simulink model "TPTC_Vehicle_dynamics_pedal2torque_NeglectSOC"  (R2026a)
settings: Solver=ode23tb  StopTime=40
model workspace (MAT data in the model file):
  BattChrgMax = -500000
  BattDischrgMax = 500000
  ChrgLmt_bpt = [1 1 1 1 1 1 1 1 0.7 0.35 0]
  DischrgLmt_bpt = [0 0.35 0.7 1 1 1 1 1 1 1 1]
  SOC_bpt = [0 10 20 30 40 50 60 70 80 90 100]
  motorMaxTorqueNm = [500 500 500 500 500 500 416.666666667 357.142857143 312.5 277.777777778 250 227.272727273 ... (16 elements, 1x16)]
  motorSpeedRadPs = [0 40 80 120 160 200 240 280 320 360 400 440 ... (16 elements, 1x16)]
values from neighbouring files (symbols this model uses):
  alpha_thr = Simulink.Parameter(300)    [init_MCU_ASR_params_only.m]
  eta_drv = Simulink.Parameter(0.95)    [init_MCU_ASR_params_only.m]
  gear_ratio_F = Simulink.Parameter(10.91)    [init_MCU_ASR_params_only.m]
  gear_ratio_R = Simulink.Parameter(11.62)    [init_MCU_ASR_params_only.m]
  J_axle = Simulink.Parameter(2*I_tire)    [init_MCU_ASR_params_only.m]
  Kd_damp = Simulink.Parameter(0.025)    [init_MCU_ASR_params_only.m]
  R_tire = Simulink.Parameter(r)    [init_MCU_ASR_params_only.m]
  T_active = Simulink.Parameter(15)    [init_MCU_ASR_params_only.m]
  T_damp_lim = Simulink.Parameter(18)    [init_MCU_ASR_params_only.m]
  tau_lpf_damp = Simulink.Parameter(0.060)    [init_MCU_ASR_params_only.m]
  Tlim_down_rate = Simulink.Parameter(2000)    [init_MCU_ASR_params_only.m]
  Tlim_up_rate = Simulink.Parameter(120)    [init_MCU_ASR_params_only.m]
  Tlim_warn_rate = Simulink.Parameter(600)    [init_MCU_ASR_params_only.m]
  Tmax_mot = Simulink.Parameter(Tn_motor)    [init_MCU_ASR_params_only.m]
  Ts_asr = Simulink.Parameter(0.001)    [init_MCU_ASR_params_only.m]
undefined symbols (not defined in the file or in its folder): dspblkCoreblockFVToolHelper, gcbh, gear_ratio
libraries: autolibsharedcoupling x8, simulink x3, autolibshareddiff x2, autolibmappedmotor x2, slpidlib x1, autolibdatasheetbattery x1, sim3dlib x1, sim3dautolib x1, vehdynlibsteering x1
(part 4 of 4)

== matlab function TPTC_Vehicle_dynamics_pedal2torque_NeglectSOC/Powertrain/03_MCU_TPTC_Controller/Slip_Detector_Front/MATLAB Function ==
  data: Te input; risk output; warn output; alpha input; Tload input; omega input; Te_opp input; alpha_opp input; Tload_opp input; omega_opp input; T_active input; alpha_thr input; state output; Ts input; Treq input; load_ratio output; follow_bad output; axis_diverge output; startup_guard output; limit_ratio output
function [risk,warn,state,load_ratio,follow_bad,...
    axis_diverge,startup_guard,limit_ratio] = f( ...
    Te,alpha,Tload,omega, ...
    Te_opp,alpha_opp,Tload_opp,omega_opp, ...
    T_active,alpha_thr,Ts,Treq)
%#codegen

% ============================================================
% MCU级 TPTC/ASR 滑移风险检测状态机
%
% 不使用滑移率，不使用车辆纵向速度。
%
% 输入：
%   Te          本轴实际/估算电机扭矩，N*m
%   alpha       本轴电机机械角加速度，rad/s^2
%   Tload       本轴电机侧负载转矩观测值，N*m
%   omega       本轴电机机械角速度，rad/s
%
%   Te_opp      对轴电机扭矩，N*m
%   alpha_opp   对轴电机角加速度，rad/s^2
%   Tload_opp   对轴负载转矩观测值，N*m
%   omega_opp   对轴电机机械角速度，rad/s
%
%   T_active    有效驱动请求阈值，N*m
%   alpha_thr   基础角加速度阈值，rad/s^2
%   Ts          控制周期，s
%   Treq        限扭前VCU目标扭矩，N*m
%
% 输出：
%   risk           Risk标志
%   warn           Warning标志
%   state          0 Normal / 1 Warning / 2 Risk
%   load_ratio     当前负载支持能力，正常约为1
%   follow_bad     负载传递异常
%   axis_diverge   前后轴动态分化诊断
%   startup_guard  起步保护标志
%   limit_ratio    目标限扭比例
%
% 状态控制：
%   Normal  ：limit_ratio = 1.00
%   Warning ：limit_ratio = 0.82
%   Risk    ：limit_ratio = 0.50~0.70，自适应
%
% 关键修改：
%   1. 持续严重负载缺失可以直接进入Risk；
%   2. 不再强制要求Risk必须伴随明显alpha异常；
%   3. Warning状态真正执行82%轻度限扭；
%   4. Warning期间负载能力仍严重不足时升级Risk；
%   5. Risk/Warning期间冻结正常负载基线；
%   6. 进入和退出均设置计数确认，避免抖振。
% ============================================================


%% ============================================================
% 1. 持久变量
% =============================================================

persistent initialized
persistent state_z

persistent active_cnt
persistent baseline_cnt
persistent baseline_valid
persistent cooldown_cnt

persistent q_fast_z
persistent q_ref_z
persistent q_rate_z

persistent omega_z
persistent omega_opp_z

persistent risk_enter_cnt
persistent warn_enter_cnt
persistent risk_reenter_cnt
persistent severe_load_cnt

persistent state_hold_cnt
persistent stable_cnt

persistent risk_ratio_z


%% ============================================================
% 2. 初始化
% =============================================================

if isempty(initialized)

    state_z = 0.0;

    active_cnt = 0.0;
    baseline_cnt = 0.0;
    baseline_valid = false;
    cooldown_cnt = 0.0;

    q_fast_z = 0.0;
    q_ref_z = 0.0;
    q_rate_z = 0.0;

    omega_z = 0.0;
    omega_opp_z = 0.0;

    risk_enter_cnt = 0.0;
    warn_enter_cnt = 0.0;
    risk_reenter_cnt = 0.0;
    severe_load_cnt = 0.0;

    state_hold_cnt = 0.0;
    stable_cnt = 0.0;

    risk_ratio_z = 0.60;

    initialized = true;
end


%% ============================================================
% 3. 采样周期和输入保护
% =============================================================

if Ts > 0.0
    Ts_eff = Ts;
else
    Ts_eff = 1.0e-3;
end

T_active_eff = max(abs(T_active),1.0);
alpha_thr_eff = max(abs(alpha_thr),1.0);

Treq_abs = abs(Treq);
Te_abs = abs(Te);
Tload_abs = abs(Tload);


%% ============================================================
% 4. 统一角加速度方向
%
% alpha_drv > 0表示电机转速幅值增加。
% =============================================================

drive_dir = 1.0;

if abs(omega) > 1.0

    if omega < 0.0
        drive_dir = -1.0;
    end

elseif Te_abs > 1.0

    if Te < 0.0
        drive_dir = -1.0;
    end
end

alpha_drv = drive_dir*alpha;


drive_dir_opp = 1.0;

if abs(omega_opp) > 1.0

    if omega_opp < 0.0
        drive_dir_opp = -1.0;
    end

elseif abs(Te_opp) > 1.0

    if Te_opp < 0.0
        drive_dir_opp = -1.0;
    end
end

alpha_opp_drv = drive_dir_opp*alpha_opp;


%% ============================================================
% 5. 标定参数
% =============================================================

% 起步保护
startup_guard_time = 0.050;
initial_blank_time = 0.050;

startup_guard_steps = ...
    max(1.0,ceil(startup_guard_time/Ts_eff));

initial_blank_steps = ...
    max(1.0,ceil(initial_blank_time/Ts_eff));


% 正常负载基线学习时间
baseline_learn_time = 0.400;

baseline_learn_steps = ...
    max(1.0,ceil(baseline_learn_time/Ts_eff));


% 回到Normal后的检测冷却时间
cooldown_time = 0.300;

cooldown_steps = ...
    max(1.0,ceil(cooldown_time/Ts_eff));


% Normal状态进入确认
risk_enter_time = 0.008;
warn_enter_time = 0.020;

risk_enter_steps = ...
    max(1.0,ceil(risk_enter_time/Ts_eff));

warn_enter_steps = ...
    max(1.0,ceil(warn_enter_time/Ts_eff));


% Warning重新升级Risk确认
risk_reenter_time = 0.020;

risk_reenter_steps = ...
    max(1.0,ceil(risk_reenter_time/Ts_eff));


% 持续严重负载不足确认
severe_load_time = 0.030;

severe_load_steps = ...
    max(1.0,ceil(severe_load_time/Ts_eff));


% Risk保持和退出确认
risk_hold_time = 0.250;
risk_stable_time = 0.200;

risk_hold_steps = ...
    max(1.0,ceil(risk_hold_time/Ts_eff));

risk_stable_steps = ...
    max(1.0,ceil(risk_stable_time/Ts_eff));


% Warning保持和退出确认
warn_hold_time = 0.300;
warn_stable_time = 0.300;

warn_hold_steps = ...
    max(1.0,ceil(warn_hold_time/Ts_eff));

warn_stable_steps = ...
    max(1.0,ceil(warn_stable_time/Ts_eff));


% 负载指标滤波
tau_q_fast = 0.030;
tau_q_ref = 1.500;
tau_q_rate = 0.030;

a_q_fast = ...
    Ts_eff/(tau_q_fast + Ts_eff);

a_q_ref = ...
    Ts_eff/(tau_q_ref + Ts_eff);

a_q_rate = ...
    Ts_eff/(tau_q_rate + Ts_eff);


% Normal状态负载阈值
q_warn_thr = 0.85;
q_risk_thr = 0.68;
q_dynamic_thr = 0.78;

% 严重负载支持能力阈值
severe_load_thr = 0.72;

% 相对负载下降速率阈值，单位1/s
q_rate_warn_thr = -0.30;
q_rate_risk_thr = -0.70;


% Risk恢复到Warning
support_risk_recover_thr = 0.80;

% Warning恢复期间重新恶化
support_reenter_thr = 0.72;

% Warning退出到Normal
support_normal_thr = 0.88;


% 角加速度阈值
alpha_warn_thr = 0.55*alpha_thr_eff;
alpha_risk_thr = 0.85*alpha_thr_eff;
alpha_strong_thr = 1.25*alpha_thr_eff;


% 限扭比例
warning_limit_ratio = 0.82;

risk_ratio_min = 0.50;
risk_ratio_max = 0.70;
risk_ratio_margin = 0.10;


% 前后轴分化阈值，仅作诊断
alpha_diff_thr = 0.60*alpha_thr_eff;
omega_diff_thr = 10.0;
omega_diff_rate_thr = 80.0;


%% ============================================================
% 6. 有效驱动请求判断
%
% 必须使用限扭前Treq。
% =============================================================

active = (Treq_abs > T_active_eff);

if active

    active_cnt = active_cnt + 1.0;

else

    active_cnt = 0.0;

    state_z = 0.0;

    baseline_cnt = 0.0;
    baseline_valid = false;
    cooldown_cnt = 0.0;

    risk_enter_cnt = 0.0;
    warn_enter_cnt = 0.0;
    risk_reenter_cnt = 0.0;
    severe_load_cnt = 0.0;

    state_hold_cnt = 0.0;
    stable_cnt = 0.0;

    risk_ratio_z = 0.60;
end

startup_guard = ...
    active && (active_cnt <= startup_guard_steps);

initial_blank = ...
    active && (active_cnt <= initial_blank_steps);


%% ============================================================
% 7. 实际扭矩执行比例
% =============================================================

if Treq_abs > 1.0

    torque_ratio_applied = ...
        Te_abs/Treq_abs;

else

    torque_ratio_applied = 0.0;
end

if torque_ratio_applied < 0.0

    torque_ratio_applied = 0.0;

elseif torque_ratio_applied > 1.20

    torque_ratio_applied = 1.20;
end


%% ============================================================
% 8. 负载观测有效性
% =============================================================

observer_valid = ...
    active && ...
    (Te_abs > max(0.20*Treq_abs,...
                  0.50*T_active_eff));


%% ============================================================
% 9. 负载指标
%
% q = |Tload_hat|/|Treq|
%
% 使用限扭前请求作分母，避免限扭动作直接改变分母。
% =============================================================

q_raw = ...
    Tload_abs/max(Treq_abs,1.0);

if q_raw < 0.0

    q_raw = 0.0;

elseif q_raw > 2.50

    q_raw = 2.50;
end


%% ============================================================
% 10. 当前负载快速滤波及变化率
% =============================================================

if ~active

    q_fast_z = q_raw;
    q_ref_z = q_raw;
    q_rate_z = 0.0;

elseif observer_valid

    if active_cnt <= 1.0

        q_fast_z = q_raw;
        q_ref_z = q_raw;
        q_rate_z = 0.0;

    else

        q_fast_old = q_fast_z;

        q_fast_z = ...
            q_fast_z + ...
            a_q_fast*(q_raw-q_fast_z);

        q_rate_raw = ...
            (q_fast_z-q_fast_old)/Ts_eff;

        q_rate_z = ...
            q_rate_z + ...
            a_q_rate*(q_rate_raw-q_rate_z);
    end

else

    % 观测无效时，变化率缓慢回零
    q_rate_z = ...
        q_rate_z + ...
        a_q_rate*(0.0-q_rate_z);
end


%% ============================================================
% 11. 冷却计数
% =============================================================

if cooldown_cnt > 0.0
    cooldown_cnt = cooldown_cnt-1.0;
end


%% ============================================================
% 12. 正常负载基线学习
%
% 只允许在：
%   Normal、基本全扭矩、动态稳定时更新。
% Warning/Risk期间冻结。
% =============================================================

normal_baseline_condition = ...
    active && ...
    observer_valid && ...
    (state_z == 0.0) && ...
    (torque_ratio_applied > 0.92) && ...
    (abs(alpha_drv) < 0.35*alpha_thr_eff);


if normal_baseline_condition

    if ~baseline_valid

        baseline_cnt = baseline_cnt + 1.0;

        if baseline_cnt <= 1.0

            q_ref_z = q_fast_z;

        else

            q_ref_z = ...
                q_ref_z + ...
                a_q_ref*(q_fast_z-q_ref_z);
        end

        if baseline_cnt >= baseline_learn_steps
            baseline_valid = true;
        end

    else

        q_ref_pre = max(q_ref_z,0.02);

        q_full_pre = ...
            q_fast_z/q_ref_pre;

        q_rate_pre = ...
            q_rate_z/q_ref_pre;

        normal_for_update = ...
            (q_full_pre > 0.90) && ...
            (q_full_pre < 1.12) && ...
            (abs(q_rate_pre) < 0.12);

        if normal_for_update

            q_ref_z = ...
                q_ref_z + ...
                a_q_ref*(q_fast_z-q_ref_z);
        end
    end
end


%% ============================================================
% 13. 负载能力指标
%
% q_full：
%   当前负载相对全扭矩正常基线的比例。
%
% q_support：
%   对当前限扭比例补偿后的负载支持能力。
% =============================================================

if baseline_valid

    q_ref_den = max(q_ref_z,0.02);

    q_full = ...
        q_fast_z/q_ref_den;

    q_rate_rel = ...
        q_rate_z/q_ref_den;

    applied_ratio_den = ...
        max(torque_ratio_applied,0.20);

    q_support = ...
        q_fast_z/...
        (q_ref_den*applied_ratio_den);

else

    q_full = 1.0;
    q_rate_rel = 0.0;
    q_support = 1.0;
end


if q_full < 0.0

    q_full = 0.0;

elseif q_full > 3.0

    q_full = 3.0;
end


if q_support < 0.0

    q_support = 0.0;

elseif q_support > 3.0

    q_support = 3.0;
end


% 对外输出当前扭矩水平下的负载支持能力
load_ratio = q_support;


%% ============================================================
% 14. Normal状态检测器使能
% =============================================================

detector_armed = ...
    baseline_valid && ...
    active && ...
    (state_z == 0.0) && ...
    (cooldown_cnt <= 0.0) && ...
    (torque_ratio_applied > 0.90);


%% ============================================================
% 15. 一般负载异常判据
% =============================================================

load_low_warn = ...
    detector_armed && ...
    (q_full < q_warn_thr);

load_low_risk = ...
    detector_armed && ...
    (q_full < q_risk_thr);

load_drop_warn = ...
    detector_armed && ...
    (q_rate_rel < q_rate_warn_thr);

load_drop_risk = ...
    detector_armed && ...
    (q_rate_rel < q_rate_risk_thr);


%% ============================================================
% 16. 持续严重负载能力不足
%
% Normal使用q_full。
% Warning使用补偿限扭影响后的q_support。
%
% 该路径不强制要求alpha异常，用于解决：
% 开式差速器单轮空转被电机平均转速掩盖的问题。
% =============================================================

if state_z == 0.0

    severe_load_metric = q_full;

    severe_load_enable = ...
        detector_armed && ...
        (torque_ratio_applied > 0.90);

elseif state_z == 1.0

    severe_load_metric = q_support;

    severe_load_enable = ...
        active && ...
        observer_valid && ...
        (torque_ratio_applied > 0.50);

else

    severe_load_metric = q_support;
    severe_load_enable = false;
end


severe_load_raw = ...
    severe_load_enable && ...
    (severe_load_metric < severe_load_thr);


if severe_load_raw

    severe_load_cnt = severe_load_cnt + 1.0;

    if severe_load_cnt > severe_load_steps
        severe_load_cnt = severe_load_steps;
    end

else

    severe_load_cnt = 0.0;
end


severe_load_confirmed = ...
    (severe_load_cnt >= severe_load_steps);


follow_bad = ...
    load_low_warn || ...
    load_drop_warn || ...
    severe_load_confirmed || ...
    ( ...
      (state_z ~= 0.0) && ...
      (q_support < support_risk_recover_thr) ...
    );


%% ============================================================
% 17. 电机角加速度条件
% =============================================================

alpha_warn = ...
    (alpha_drv > alpha_warn_thr);

alpha_risk = ...
    (alpha_drv > alpha_risk_thr);

alpha_strong = ...
    (alpha_drv > alpha_strong_thr);


%% ============================================================
% 18. 前后轴动态分化诊断
%
% 当前仅输出诊断，不直接决定状态。
% =============================================================

omega_diff = ...
    abs(omega)-abs(omega_opp);

omega_diff_old = ...
    abs(omega_z)-abs(omega_opp_z);

d_omega_diff = ...
    (omega_diff-omega_diff_old)/Ts_eff;


alpha_diverge = ...
    (~startup_guard) && ...
    alpha_warn && ...
    (alpha_drv > ...
     alpha_opp_drv+alpha_diff_thr);


omega_diverge = ...
    (~startup_guard) && ...
    (omega_diff > omega_diff_thr) && ...
    (d_omega_diff > omega_diff_rate_thr);


axis_diverge = ...
    alpha_diverge || omega_diverge;


%% ============================================================
% 19. Normal状态进入条件
% =============================================================

risk_enter_raw = false;
warn_enter_raw = false;

if state_z == 0.0 && ...
        active && ...
        (~initial_blank)

    % 路径1：负载严重降低并伴随动态异常
    risk_path_main = ...
        load_low_risk && ...
        (alpha_risk || load_drop_risk);

    % 路径2：负载中度降低且快速恶化
    risk_path_dynamic = ...
        detector_armed && ...
        (q_full < q_dynamic_thr) && ...
        load_drop_risk && ...
        alpha_warn;

    % 路径3：极强角加速度且负载已经下降
    risk_path_strong = ...
        detector_armed && ...
        alpha_strong && ...
        (q_full < 0.90);

    % 路径4：持续严重负载不足
    % 不要求alpha必须明显异常
    risk_path_sustained_load = ...
        severe_load_confirmed;

    risk_enter_raw = ...
        risk_path_main || ...
        risk_path_dynamic || ...
        risk_path_strong || ...
        risk_path_sustained_load;


    % Warning：中度负载异常
    warn_path_main = ...
        load_low_warn && ...
        (alpha_warn || load_drop_warn);

    warn_enter_raw = ...
        warn_path_main;
end


% Risk优先
if risk_enter_raw
    warn_enter_raw = false;
end


%% ============================================================
% 20. Normal状态进入确认计数
% =============================================================

if risk_enter_raw

    risk_enter_cnt = risk_enter_cnt + 1.0;

    if risk_enter_cnt > risk_enter_steps
        risk_enter_cnt = risk_enter_steps;
    end

else

    risk_enter_cnt = 0.0;
end


if warn_enter_raw

    warn_enter_cnt = warn_enter_cnt + 1.0;

    if warn_enter_cnt > warn_enter_steps
        warn_enter_cnt = warn_enter_steps;
    end

else

    warn_enter_cnt = 0.0;
end


risk_enter = ...
    (risk_enter_cnt >= risk_enter_steps);

warn_enter = ...
    (warn_enter_cnt >= warn_enter_steps);


%% ============================================================
% 21. Warning重新升级Risk
%
% 满足任一条件：
%   1. 极强角加速度；
%   2. 持续严重负载能力不足；
%   3. 负载支持能力低且角加速度异常。
% =============================================================

risk_reenter_raw = ...
    (state_z == 1.0) && ...
    active && ...
    ( ...
      alpha_strong || ...
      severe_load_confirmed || ...
      ( ...
        (q_support < support_reenter_thr) && ...
        alpha_warn ...
      ) ...
    );


if risk_reenter_raw

    risk_reenter_cnt = risk_reenter_cnt + 1.0;

    if risk_reenter_cnt > risk_reenter_steps
        risk_reenter_cnt = risk_reenter_steps;
    end

else

    risk_reenter_cnt = 0.0;
end


risk_reenter = ...
    (risk_reenter_cnt >= risk_reenter_steps);


%% ============================================================
% 22. 三状态状态机
% =============================================================

if ~active

    % --------------------------------------------------------
    % 无驱动请求
    % --------------------------------------------------------

    state_z = 0.0;

    state_hold_cnt = 0.0;
    stable_cnt = 0.0;


elseif state_z == 0.0

    % --------------------------------------------------------
    % Normal
    % --------------------------------------------------------

    state_hold_cnt = 0.0;
    stable_cnt = 0.0;

    if risk_enter

        % 根据检测时负载能力确定Risk限扭比例
        ratio_candidate = ...
            q_full+risk_ratio_margin;

        if ratio_candidate < risk_ratio_min

            risk_ratio_z = risk_ratio_min;

        elseif ratio_candidate > risk_ratio_max

            risk_ratio_z = risk_ratio_max;

        else

            risk_ratio_z = ratio_candidate;
        end

        state_z = 2.0;

        risk_enter_cnt = 0.0;
        warn_enter_cnt = 0.0;
        risk_reenter_cnt = 0.0;
        severe_load_cnt = 0.0;

        state_hold_cnt = 0.0;
        stable_cnt = 0.0;


    elseif warn_enter

        state_z = 1.0;

        warn_enter_cnt = 0.0;
        risk_reenter_cnt = 0.0;

        state_hold_cnt = 0.0;
        stable_cnt = 0.0;
    end


elseif state_z == 2.0

    % --------------------------------------------------------
    % Risk：快速限扭
    % --------------------------------------------------------

    state_hold_cnt = state_hold_cnt + 1.0;

    if state_hold_cnt >= risk_hold_steps

        risk_stable = ...
            (q_support > support_risk_recover_thr) && ...
            (alpha_drv < 0.55*alpha_thr_eff);

        if risk_stable

            stable_cnt = stable_cnt + 1.0;

            if stable_cnt >= risk_stable_steps

                % Risk先退出到Warning
                state_z = 1.0;

                state_hold_cnt = 0.0;
                stable_cnt = 0.0;

                risk_reenter_cnt = 0.0;
                severe_load_cnt = 0.0;
            end

        else

            stable_cnt = 0.0;
        end
    end


else

    % --------------------------------------------------------
    % Warning：轻度限扭/恢复观察
    % --------------------------------------------------------

    state_hold_cnt = state_hold_cnt + 1.0;

    if risk_reenter

        % 重新恶化，根据当前执行比例再下降约10%
        ratio_candidate = ...
            torque_ratio_applied-0.10;

        if ratio_candidate < risk_ratio_min

            risk_ratio_z = risk_ratio_min;

        elseif ratio_candidate > risk_ratio_max

            risk_ratio_z = risk_ratio_max;

        else

            risk_ratio_z = ratio_candidate;
        end

        state_z = 2.0;

        state_hold_cnt = 0.0;
        stable_cnt = 0.0;

        risk_reenter_cnt = 0.0;
        severe_load_cnt = 0.0;


    elseif state_hold_cnt >= warn_hold_steps

        % Warning期间已经执行82%轻度限扭，
        % 因此不能再要求Te/Treq > 0.95，否则无法退出。
        normal_recovered = ...
            (q_support > support_normal_thr) && ...
            (abs(alpha_drv) < 0.40*alpha_thr_eff) && ...
            (~severe_load_confirmed);

        if normal_recovered

            stable_cnt = stable_cnt + 1.0;

            if stable_cnt >= warn_stable_steps

                state_z = 0.0;

                state_hold_cnt = 0.0;
                stable_cnt = 0.0;

                risk_reenter_cnt = 0.0;
                severe_load_cnt = 0.0;

                % 防止刚回Normal时恢复扭矩造成再次误触发
                cooldown_cnt = cooldown_steps;
            end

        else

            stable_cnt = 0.0;
        end
    end
end


%% ============================================================
% 23. 输出
% =============================================================

state = state_z;

risk = ...
    (state_z == 2.0);

warn = ...
    (state_z == 1.0);


if state_z == 2.0

    % Risk：自适应强限扭
    limit_ratio = risk_ratio_z;

elseif state_z == 1.0

    % Warning：82%轻度限扭
    limit_ratio = warning_limit_ratio;

else

    % Normal：不限制
    limit_ratio = 1.0;
end


%% ============================================================
% 24. 更新历史量
% =============================================================

omega_z = omega;
omega_opp_z = omega_opp;

% 当前版本保留对轴负载接口
unused_Tload_opp = Tload_opp; %#ok<NASGU>

end

== matlab function TPTC_Vehicle_dynamics_pedal2torque_NeglectSOC/Powertrain/03_MCU_TPTC_Controller/Torque_Limiter/Torque_Limiter_Front/Fast_Down_Slow_Up_Limiter ==
  data: T_req input; T_cmd_limited output; risk input; warn input; limit_ratio input; Tmax_mot parameter; Tlim_up_rate parameter; Tlim_down_rate parameter; Tlim_warn_rate input; Ts input; state output
function [T_cmd_limited,state] = f( ...
    T_req,risk,warn,limit_ratio, ...
    Tmax_mot,Tlim_up_rate,Tlim_down_rate,...
    Tlim_warn_rate,Ts)
%#codegen

% ============================================================
% MCU级三级自适应限扭器
%
% state：
%   0 Normal  ：100%
%   1 Warning ：通常82%，轻度限扭
%   2 Risk    ：50%～70%，快速限扭
%
% limit_ratio由Slip Detector给出：
%   Normal  = 1.00
%   Warning = 0.82
%   Risk    = 自适应0.50～0.70
% ============================================================

persistent initialized
persistent T_cmd_z
persistent limited_z

if isempty(initialized)

    T_cmd_z = 0.0;
    limited_z = false;

    initialized = true;
end


%% 采样周期

if Ts > 0.0
    Ts_eff = Ts;
else
    Ts_eff = 1.0e-3;
end


%% 参数保护

Tmax_eff = max(abs(Tmax_mot),1.0);

up_rate = max(abs(Tlim_up_rate),1.0);

risk_down_rate = ...
    max(abs(Tlim_down_rate),1.0);

warn_down_rate = ...
    max(abs(Tlim_warn_rate),1.0);


%% 请求扭矩

T_req_abs = min(abs(T_req),Tmax_eff);

req_sign = 1.0;

if T_req < 0.0
    req_sign = -1.0;
end


%% 状态

if risk

    state = 2.0;

elseif warn

    state = 1.0;

else

    state = 0.0;
end


%% 无扭矩请求

if T_req_abs < 0.5

    T_cmd_z = 0.0;
    limited_z = false;

    T_cmd_limited = 0.0;
    return;
end


%% 扭矩方向变化

if T_cmd_z*T_req < 0.0

    T_cmd_z = 0.0;
    limited_z = false;
end


%% 限扭比例保护

ratio_eff = limit_ratio;

if ratio_eff < 0.45

    ratio_eff = 0.45;

elseif ratio_eff > 1.0

    ratio_eff = 1.0;
end


%% 目标扭矩

T_target_abs = ...
    ratio_eff*T_req_abs;

T_current_abs = ...
    abs(T_cmd_z);


if state ~= 0.0 || ratio_eff < 0.999

    limited_z = true;
end


%% 扭矩下降

if T_target_abs < T_current_abs

    if state == 2.0

        % Risk快速下降
        step_down = ...
            risk_down_rate*Ts_eff;

        T_current_abs = ...
            max(T_target_abs,...
            T_current_abs-step_down);

    elseif state == 1.0

        % Warning中速下降
        step_down = ...
            warn_down_rate*Ts_eff;

        T_current_abs = ...
            max(T_target_abs,...
            T_current_abs-step_down);

    else

        % 上层主动降低扭矩请求时直接跟随
        T_current_abs = T_target_abs;
    end


%% 扭矩增加和恢复

elseif T_target_abs > T_current_abs

    if limited_z

        % 发生过限扭后慢速恢复
        step_up = ...
            up_rate*Ts_eff;

        T_current_abs = ...
            min(T_target_abs,...
            T_current_abs+step_up);

    else

        % 正常请求直接跟随
        T_current_abs = T_target_abs;
    end
end


%% 恢复完成

if state == 0.0 && ...
        abs(T_current_abs-T_req_abs) < 0.5

    limited_z = false;
end


%% 输出

T_cmd_z = ...
    req_sign*T_current_abs;

T_cmd_limited = T_cmd_z;

end

== matlab function TPTC_Vehicle_dynamics_pedal2torque_NeglectSOC/Powertrain/03_MCU_TPTC_Controller/Torque_Limiter/Torque_Limiter_Rear/Fast_Down_Slow_Up_Limiter ==
  data: T_req input; T_cmd_limited output; risk input; warn input; limit_ratio input; Tmax_mot parameter; Tlim_up_rate parameter; Tlim_down_rate parameter; Tlim_warn_rate input; Ts input; state output
function [T_cmd_limited,state] = f( ...
    T_req,risk,warn,limit_ratio, ...
    Tmax_mot,Tlim_up_rate,Tlim_down_rate,...
    Tlim_warn_rate,Ts)
%#codegen

% ============================================================
% MCU级三级自适应限扭器
%
% state：
%   0 Normal  ：100%
%   1 Warning ：通常82%，轻度限扭
%   2 Risk    ：50%～70%，快速限扭
%
% limit_ratio由Slip Detector给出：
%   Normal  = 1.00
%   Warning = 0.82
%   Risk    = 自适应0.50～0.70
% ============================================================

persistent initialized
persistent T_cmd_z
persistent limited_z

if isempty(initialized)

    T_cmd_z = 0.0;
    limited_z = false;

    initialized = true;
end


%% 采样周期

if Ts > 0.0
    Ts_eff = Ts;
else
    Ts_eff = 1.0e-3;
end


%% 参数保护

Tmax_eff = max(abs(Tmax_mot),1.0);

up_rate = max(abs(Tlim_up_rate),1.0);

risk_down_rate = ...
    max(abs(Tlim_down_rate),1.0);

warn_down_rate = ...
    max(abs(Tlim_warn_rate),1.0);


%% 请求扭矩

T_req_abs = min(abs(T_req),Tmax_eff);

req_sign = 1.0;

if T_req < 0.0
    req_sign = -1.0;
end


%% 状态

if risk

    state = 2.0;

elseif warn

    state = 1.0;

else

    state = 0.0;
end


%% 无扭矩请求

if T_req_abs < 0.5

    T_cmd_z = 0.0;
    limited_z = false;

    T_cmd_limited = 0.0;
    return;
end


%% 扭矩方向变化

if T_cmd_z*T_req < 0.0

    T_cmd_z = 0.0;
    limited_z = false;
end


%% 限扭比例保护

ratio_eff = limit_ratio;

if ratio_eff < 0.45

    ratio_eff = 0.45;

elseif ratio_eff > 1.0

    ratio_eff = 1.0;
end


%% 目标扭矩

T_target_abs = ...
    ratio_eff*T_req_abs;

T_current_abs = ...
    abs(T_cmd_z);


if state ~= 0.0 || ratio_eff < 0.999

    limited_z = true;
end


%% 扭矩下降

if T_target_abs < T_current_abs

    if state == 2.0

        % Risk快速下降
        step_down = ...
            risk_down_rate*Ts_eff;

        T_current_abs = ...
            max(T_target_abs,...
            T_current_abs-step_down);

    elseif state == 1.0

        % Warning中速下降
        step_down = ...
            warn_down_rate*Ts_eff;

        T_current_abs = ...
            max(T_target_abs,...
            T_current_abs-step_down);

    else

        % 上层主动降低扭矩请求时直接跟随
        T_current_abs = T_target_abs;
    end


%% 扭矩增加和恢复

elseif T_target_abs > T_current_abs

    if limited_z

        % 发生过限扭后慢速恢复
        step_up = ...
            up_rate*Ts_eff;

        T_current_abs = ...
            min(T_target_abs,...
            T_current_abs+step_up);

    else

        % 正常请求直接跟随
        T_current_abs = T_target_abs;
    end
end


%% 恢复完成

if state == 0.0 && ...
        abs(T_current_abs-T_req_abs) < 0.5

    limited_z = false;
end


%% 输出

T_cmd_z = ...
    req_sign*T_current_abs;

T_cmd_limited = T_cmd_z;

end
